simulink model "DC_Double_Closed_Loop_Speed_Regulation1"  (R2016a)
settings: Solver=VariableStepAuto  SolverMode=SingleTasking  StartTime=0  StopTime=2.5  MaxStep=1e-5  RelTol=1e-3
InitFcn:
  | run('DC_Double_Closed_Loop_Speed_Regulation.m')
values from neighbouring files (symbols this model uses):
  alpha = Un/nN    (= 0.00666666666667)    [DC_Double_Closed_Loop_Speed_Regulation.m]
  beta = Uonl/(lambda*IdN)    [DC_Double_Closed_Loop_Speed_Regulation.m]
  Ce = 0.1459    [DC_Double_Closed_Loop_Speed_Regulation.m]
  Ki = KI*taui*R/(Ks*beta)    [DC_Double_Closed_Loop_Speed_Regulation.m]    (also in motor.m = 0.5)
  Kn = (h+1)*beta*Ce*Tm/(2*h*alpha*R*Tsigman)    [DC_Double_Closed_Loop_Speed_Regulation.m]
  R = 3.68    [DC_Double_Closed_Loop_Speed_Regulation.m]    (also in motor.m = 1)
  taui = Tl    (= 0.0144)    [DC_Double_Closed_Loop_Speed_Regulation.m]
  taun = h*Tsigman    (= 0.05625)    [DC_Double_Closed_Loop_Speed_Regulation.m]
  Tl = 0.0144    [DC_Double_Closed_Loop_Speed_Regulation.m]
  Tm = 0.18    [DC_Double_Closed_Loop_Speed_Regulation.m]
  Toi = 0.0005    [DC_Double_Closed_Loop_Speed_Regulation.m]
  Ton = 0.01    [DC_Double_Closed_Loop_Speed_Regulation.m]
  Ts = 1/f    (= 0.000125)    [DC_Double_Closed_Loop_Speed_Regulation.m]
  Ucm = 5    [DC_Double_Closed_Loop_Speed_Regulation.m]
  Un = 10    [DC_Double_Closed_Loop_Speed_Regulation.m]
  Uoil = 5    [DC_Double_Closed_Loop_Speed_Regulation.m]
  Uonl = 10    [DC_Double_Closed_Loop_Speed_Regulation.m]
undefined symbols (not defined in the file or in its folder): powergui
libraries: powerlib x7, powerlib_meascontrol x1, simulink x1
settings Model: Creator=ywtyfp  LastModifiedBy=Administrator
settings DataIOCC: ReturnWorkspaceOutputs=on
settings DebuggingCC: SFUnexpectedBacktrackingDiag=error  SFNoUnconditionalDefaultTransitionDiag=error
settings SFSimCC: SimUseLocalCustomCode=on
settings RTWCC: RTWUseLocalCustomCode=on
settings GRTTargetCC: TargetLangStandard=C99 (ISO)
settings ConfigComp: CovMetricSettings=dwe  CovHtmlReporting=off  CovSaveCumulativeToWorkspaceVar=off  CovSaveSingleToWorkspaceVar=off  CovExternalEMLEnable=on

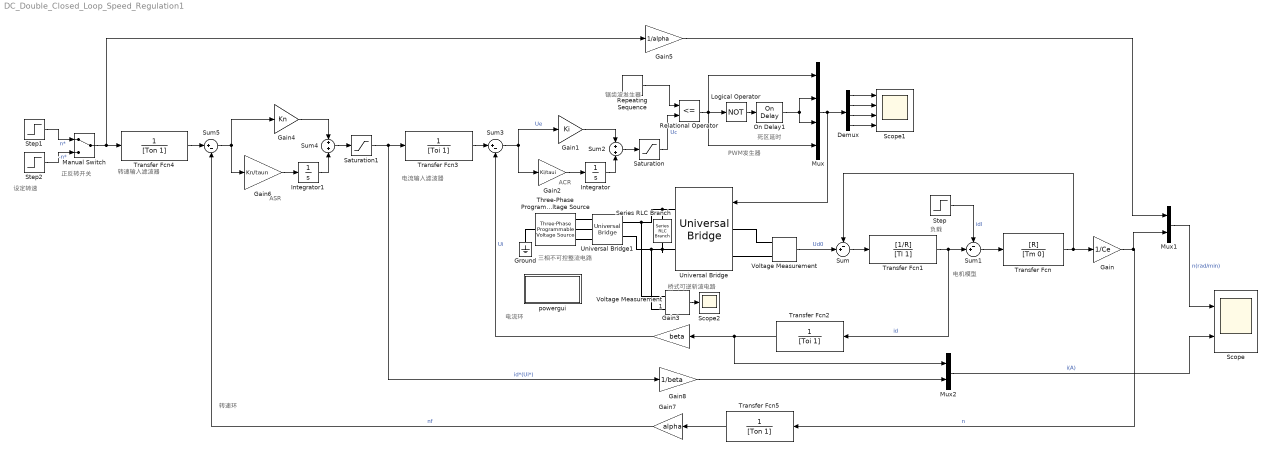
== system DC_Double_Closed_Loop_Speed_Regulation1 ==
  note: 设定转速
  note: 电流环
  note: 转速环
  note: 转速输入滤波器
  note: ASR
  note: ACR
  note: 电流输入滤波器
  note: 负载
  note: 电机模型
  note: PWM发生器
  note: 桥式可逆斩波电路
  note: 锯齿波发生器
  note: 死区延时
  note: 正反转开关
  note: 三相不可控整流电路
  Demux : Demux
  Gain : Gain  Gain=1/Ce
  Gain1 : Gain  Gain=Ki
  Gain2 : Gain  Gain=Ki/taui
  Gain3 : Gain  Gain=beta
  Gain4 : Gain  Gain=Kn
  Gain5 : Gain  Gain=1/alpha
  Gain6 : Gain  Gain=Kn/taun
  Gain7 : Gain  Gain=alpha
  Gain8 : Gain  Gain=1/beta
  Ground : powerlib/Elements/Ground  LConnTagsString=a
  Integrator : Integrator  LimitOutput=on  UpperSaturationLimit=Uoil  LowerSaturationLimit=-Uoil
  Integrator1 : Integrator  LimitOutput=on  UpperSaturationLimit=Uonl  LowerSaturationLimit=-Uonl
  Logical Operator : Logic  Operator=NOT  AllPortsSameDT=off  OutDataTypeStr=boolean
  Manual Switch : ManualSwitch
  Mux : Mux
  Mux1 : Mux  Inputs=2
  Mux2 : Mux  Inputs=2
  On Delay1 : powerlib_meascontrol/Logic/On Delay  DelayType=On delay  delay=3e-6  ic=0  Ts=0
  Relational Operator : RelationalOperator  Operator=<=  OutDataTypeStr=boolean
  Repeating Sequence : simulink/Sources/Repeating Sequence  rep_seq_t=[0 Ts]  rep_seq_y=[-Ucm Ucm]
  Saturation : Saturate  UpperLimit=Uoil  LowerLimit=-Uoil
  Saturation1 : Saturate  UpperLimit=Uonl  LowerLimit=-Uonl
  Scope : Scope  NumInputPorts=2
  Scope1 : Scope  NumInputPorts=4
  Scope2 : Scope
  Series RLC Branch : powerlib/Elements/Series RLC Branch  LConnTagsString=__new0  RConnTagsString=__new0  BranchType=C  Resistance=1  Inductance=1e-3  SetiL0=off  InitialCurrent=0  Capacitance=1e-4  Setx0=off  InitialVoltage=0  Measurements=None
  Step : Step  Time=0  After=0  SampleTime=0
  Step1 : Step  Time=0.1  After=Un  SampleTime=0
  Step2 : Step  Time=0.1  After=-Un  SampleTime=0
  Sum : Sum  Inputs=-+|
  Sum1 : Sum  Inputs=-+|
  Sum2 : Sum  Inputs=+|+
  Sum3 : Sum  Inputs=|+-
  Sum4 : Sum  Inputs=+|+
  Sum5 : Sum  Inputs=|+-
  Three-Phase Programmable Voltage Source : powerlib/Electrical Sources/Three-Phase Programmable Voltage Source  PositiveSequence="[380  0 50]"  VariationEntity=None  VariationType=Table of time-amplitude pairs  VariationTypeAlt=Step  VariationStep=0.5  VariationRate=10  VariationMagnitude=0.3  VariationFrequency=2  VariationTiming=[1 2]  VariationPhaseA=off  Amplitudes=[1 0.8 1.2 1.0]  TimeValues=[0 0.1 0.15 0.2]  HarmonicGeneration=off  HarmonicA=[3 0.2 -25 0]  HarmonicB=[2 0.15 35 2]  Timing="[0.05  3]"  BusType=swing  Pref=0  Qref=0  Qmin=-inf  Qmax=inf
  Transfer Fcn : TransferFcn  Numerator=[R]  Denominator=[Tm 0]
  Transfer Fcn1 : TransferFcn  Numerator=[1/R]  Denominator=[Tl 1]
  Transfer Fcn2 : TransferFcn  Denominator=[Toi 1]
  Transfer Fcn3 : TransferFcn  Denominator=[Toi 1]
  Transfer Fcn4 : TransferFcn  Denominator=[Ton 1]
  Transfer Fcn5 : TransferFcn  Denominator=[Ton 1]
  Universal Bridge : powerlib/Power Electronics/Universal Bridge  Arms=2  SnubberResistance=1e5  SnubberCapacitance=inf  Device=IGBT / Diodes  Ron=1e-3  Lon=0  ForwardVoltages="[  0  0  ]"  ForwardVoltage=0  GTOparameters=[ 10e-6 , 20e-6 ]  IGBTparameters=[ 1e-6 , 2e-6 ]  Measurements=None  Measurements_2=None  converterType=Rectifier
  Universal Bridge1 : powerlib/Power Electronics/Universal Bridge  Arms=3  SnubberResistance=1e5  SnubberCapacitance=inf  Device=Diodes  Ron=1e-3  Lon=0  ForwardVoltages="[  0  0  ]"  ForwardVoltage=0  GTOparameters=[ 10e-6 , 20e-6 ]  IGBTparameters=[ 1e-6 , 2e-6 ]  Measurements=None  Measurements_2=None  converterType=Rectifier
  Voltage Measurement : powerlib/Measurements/Voltage Measurement  PhasorSimulation=off  OutputType=Complex  PSBequivalent=0
  Voltage Measurement1 : powerlib/Measurements/Voltage Measurement  PhasorSimulation=off  OutputType=Complex  PSBequivalent=0
  powergui : Subsystem  Priority=1  AncestorBlock=powerlib/powergui  DialogController=POWERSYS.PowerSysDialog  InitFcn=powergui( 'InitFcn_Callback' , gcb , 0 , [ ] );  mask(PSB option menu block){SimulationMode=Continuous, SampleTime=50e-6, frequency=60, Iterations=50, frequencyindice=50, Pbase=100e6, ErrMax=1e-4, UnitsV=kV, UnitsW=MW, buscounter=0, FunctionMessages=off, echomessages=off, EnableUseOfTLC=off, CurrentSourceSwitches=off, DisableSnubberDevices=off, DisableRonSwitches=off, DisableVfSwitches=off, DisplayEquations=off, AutomaticDiscreteSolvers=off, SolverType=Tustin/Backward Euler (TBE), Interpol=off, ExternalGateDelay=off, methode=off, Ts=100, x0status=blocks, SPID=on, SwTol=0, HookPort=off, NonlinearTolerance=1e-4, nMaxIteration=100, ContinueOnMaxIteration=off, RestoreLinks=warning, ResistiveCurrentMeasurement=off, Frange=[0:2:500], Ylog=off, Xlog=on, ShowGrid=off, save=off, variable=ZData, structure=0, ZoomFFT=off, StartTime=0.0, cycles=1, DisplayStyle=1, fundamental=60, FreqAxis=off, MaxFrequency=1000, frequencyindicesteady=1, RmsSteady=1, display=off}
      mask prompts: SimulationMode "Simulation type:"; SampleTime "Sample time (s):"; frequency "Frequency (Hz):"; Iterations "Max iterations"; frequencyindice "Frequency (Hz)"; Pbase "Base power (VA)"; ErrMax "PQ tolerance (pu)"; UnitsV "Voltage units"; UnitsW "Power units"; buscounter "Load flow bus counter"; FunctionMessages "Disable Specialized Power Systems warnings"; echomessages "Display Specialized Power Systems compilation messages"; EnableUseOfTLC "Use TLC file when in Accelerator Simulation Mode and for code generation"; CurrentSourceSwitches "Disable ideal switching"; DisableSnubberDevices "Disable snubbers in switching devices"; DisableRonSwitches "Disable Ron resistances in switching devices"; DisableVfSwitches "Disable forward voltages in switching devices"; DisplayEquations "Display circuit differential equations"; AutomaticDiscreteSolvers "Automatically handle Discrete solver and Advanced tab solver settings of blocks"; SolverType "Discrete solver"; Interpol "Interpolate switching events"; ExternalGateDelay "Use time-stamped gate signals"; methode "Store switching topologies"; Ts "Buffer size (MBytes):"; x0status "Start simulation with initial electrical states from:"; SPID "Use ideal switching devices"; SwTol "Switch tolerance"; HookPort "Allow multiple powergui blocks"; NonlinearTolerance "Solver tolerance"; nMaxIteration "Maximum number of iterations"; ContinueOnMaxIteration "Continue Simulation if maximum number of iterations is reached"; RestoreLinks "Restore disabled links of Simscape Power Systems ST blocks:"; ResistiveCurrentMeasurement "Use non ideal current measurement blocks (1e-4Ohm internal resistance)"; Frange "Frequency Range"; Ylog "Log impedance"; Xlog "log Frequency"; ShowGrid "grid"; save "Save Data To Workspace"; variable "Variable Name"; structure "Structure Name (PSBFFTSCOPE)"; ZoomFFT "ZoomFFT (PSBFFTSCOPE)"; StartTime "Start Time (PSBFFTSCOPE)"; cycles "Cycles (PSBFFTSCOPE)"; DisplayStyle "Display style (PSBFFTSCOPE)"; fundamental "Fundamental (PSBFFTSCOPE)"; FreqAxis "Frequency Axis (PSBFFTSCOPE)"; MaxFrequency "Max Frequency (PSBFFTSCOPE)"; frequencyindicesteady "Frequency indice (STEADYSTATE)"; RmsSteady "RMS display (STEADYSTATE)"; display "Display Results"
      mask help: Set simulation type, simulation parameters, and preferences.
      mask init:
      | dispMessage = powergui('MaskInitialization',gcb,SimulationMode,SampleTime);
      settings: PreSaveFcn=powergui( 'PreSaveFcn_Callback' , gcb , [ ] , [ ] );  OpenFcn=sps_rtmsupport('OpenFcn',gcbh)
      mask Help: helpview(psbhelp)
      mask TypeOptions SimulationMode: Continuous | Discrete | Phasor | Discrete phasor
      mask Callback SimulationMode: powergui('SimulationType',[],[],gcb);
      mask TypeOptions UnitsV: V | kV
      mask TypeOptions UnitsW: W | kW | MW
      mask Callback CurrentSourceSwitches: powergui('SimulationType',[],[],gcb);
      mask Callback AutomaticDiscreteSolvers: powergui('SimulationType',[],[],gcb);
      mask TypeOptions SolverType: Tustin/Backward Euler (TBE) | Tustin | Backward Euler
      mask Callback SolverType: powergui('SimulationType',[],[],gcb);
      mask Callback Interpol: powergui('SimulationType',[],[],gcb);
      mask Callback ExternalGateDelay: powergui('SimulationType',[],[],gcb);
      mask Callback methode: powergui('SimulationType',[],[],gcb);
      mask TypeOptions x0status: blocks | steady | zero
      mask TypeOptions RestoreLinks: yes | warning | no
      mask Callback display: sps_rtmsupport('parametereditingmodes',gcbh) % Will be executed last in parameter callbacks to ensure mask enable consistency
      mask DialogControl AutoSolverNote Prompt: The Simulation type parameter is governed by Simulink. To access the Powergui solver settings, unselect auto (Automatic solver selection) solver in the Simulink solver options.
      mask DialogControl SteadyState Prompt: Steady-State
      mask DialogControl SteadyState Callback:
      | close_system(gcb)
      | power_steadystate(bdroot(gcb),gcb);
      mask DialogControl InitialState Prompt: Initial State
      mask DialogControl InitialState Callback:
      | close_system(gcb)
      | power_initstates(bdroot(gcb),gcb)
      mask DialogControl MachineInitialization Prompt: Machine Initialization
      mask DialogControl MachineInitialization Callback:
      | close_system(gcb)
      | power_loadflow(bdroot(gcb),gcb)
      mask DialogControl ImpedanceMeasurement Prompt: Impedance Measurement
      mask DialogControl ImpedanceMeasurement Callback:
      | close_system(gcb)
      | power_zmeter(bdroot(gcb),gcb)
      mask DialogControl FFTAnalysis Prompt: FFT Analysis
      mask DialogControl FFTAnalysis Callback:
      | close_system(gcb)
      | power_fftscope(bdroot(gcb),gcb)
      mask DialogControl LinearSystemAnalyzer Prompt: Use Linear System Analyzer
      mask DialogControl LinearSystemAnalyzer Callback:
      | close_system(gcb)
      | power_ltiview(bdroot(gcb),gcb)
      mask DialogControl HysteresisDesign Prompt: Hysteresis Design
      mask DialogControl HysteresisDesign Callback:
      | close_system(gcb)
      | power_hysteresis(bdroot(gcb),gcb)
      mask DialogControl RLCLineParameters Prompt: RLC Line Parameters
      mask DialogControl RLCLineParameters Callback:
      | close_system(gcb)
      | power_lineparam(bdroot(gcb),gcb)
      mask DialogControl GenerateReprot Prompt: Generate Report
      mask DialogControl GenerateReprot Callback:
      | close_system(gcb)
      | power_report(bdroot(gcb),gcb)
      mask DialogControl Control14 Prompt: Customize SPS blocks
      mask DialogControl Control14 Callback:
      | close_system(gcb);
      | power_customize;
      mask DialogControl LoadFlow Prompt: Load Flow
      mask DialogControl LoadFlow Callback:
      | close_system(gcb)
      | power_loadflow('-v2',bdroot(gcb))
      mask DialogControl Container14 Prompt: Load flow settings
      mask DialogControl Solver Prompt: Solver
      mask DialogControl SolverDetails Prompt: Solver details for nonlinear elements
      mask Display: color('blue'),disp(dispMessage)
  wires:
  Sum/1 -> Transfer Fcn1/1
  Sum1/1 -> Transfer Fcn/1
  Transfer Fcn/1 -> Sum/1, Gain/1
  Gain/1 -> Mux1/2, Transfer Fcn5/1  "n"
  Step/1 -> Sum1/1  "idl"
  Voltage Measurement/1 -> Sum/2  "Ud0"
  Repeating Sequence/1 -> Relational Operator/1
  Mux/1 -> Demux/1, Universal Bridge/1
  Gain2/1 -> Integrator/1
  Saturation/1 -> Relational Operator/2  "Uc"
  Integrator/1 -> Sum2/2
  Sum2/1 -> Saturation/1
  Gain1/1 -> Sum2/1
  Transfer Fcn2/1 -> Mux2/1, Gain3/1
  Transfer Fcn1/1 -> Transfer Fcn2/1, Sum1/2  "id"
  Gain3/1 -> Sum3/2  "Ui"
  Sum3/1 -> Gain2/1, Gain1/1  "Ue"
  Transfer Fcn3/1 -> Sum3/1
  Gain4/1 -> Sum4/1
  Sum4/1 -> Saturation1/1
  Integrator1/1 -> Sum4/2
  Gain6/1 -> Integrator1/1
  Saturation1/1 -> Transfer Fcn3/1, Gain8/1  "id*(Ui*)"
  Transfer Fcn5/1 -> Gain7/1
  Gain7/1 -> Sum5/2  "nf"
  Sum5/1 -> Gain6/1, Gain4/1
  Transfer Fcn4/1 -> Sum5/1
  Mux1/1 -> Scope/1  "n(rad/min)"
  Gain5/1 -> Mux1/1
  Mux2/1 -> Scope/2  "i(A)"
  Relational Operator/1 -> Mux/4, Mux/1, Logical Operator/1
  Demux/3 -> Scope1/3
  Demux/4 -> Scope1/4
  Demux/2 -> Scope1/2
  Demux/1 -> Scope1/1
  Logical Operator/1 -> On Delay1/1
  Gain8/1 -> Mux2/2
  Voltage Measurement1/1 -> Scope2/1
  On Delay1/1 -> Mux/2, Mux/3
  Manual Switch/1 -> Gain5/1, Transfer Fcn4/1
  Step1/1 -> Manual Switch/1  "n*"
  Step2/1 -> Manual Switch/2  "-n*"
  connections:
  Universal Bridge1/RConn1 -- Series RLC Branch/LConn1 -- Universal Bridge/RConn1 -- Voltage Measurement1/LConn1
  Universal Bridge1/RConn2 -- Voltage Measurement1/LConn2 -- Series RLC Branch/RConn1 -- Universal Bridge/RConn2
  Universal Bridge/LConn1 -- Voltage Measurement/LConn1
  Universal Bridge/LConn2 -- Voltage Measurement/LConn2
  Three-Phase Programmable Voltage Source/LConn1 -- Ground/LConn1
  Three-Phase Programmable Voltage Source/RConn3 -- Universal Bridge1/LConn3
  Three-Phase Programmable Voltage Source/RConn2 -- Universal Bridge1/LConn2
  Three-Phase Programmable Voltage Source/RConn1 -- Universal Bridge1/LConn1

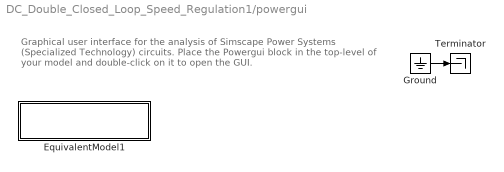
== system DC_Double_Closed_Loop_Speed_Regulation1/powergui ==
  note: Graphical user interface for the analysis of
      | Simscape Power Systems (Specialized Technology) circuits.
      | Place the Powergui block in the top-level of your model and double-click
      | on it to open the GUI.
  EquivalentModel1 : Subsystem  mask{SwTol=SwTol}
      mask prompts: SwTol "SwitchTolerance"
      mask init:
      | S  = GetDataForEquivalentModel('SPID',gcbh,SwTol);
      mask Display:
      | color('blue')
      | disp('EQUIVALENT CIRCUIT\nSPID')
  Ground : Ground
  Terminator : Terminator
  wires:
  Ground/1 -> Terminator/1

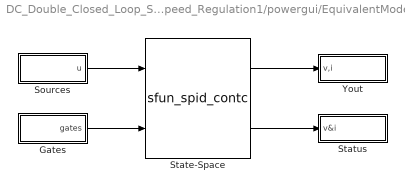
== system DC_Double_Closed_Loop_Speed_Regulation1/powergui/EquivalentModel1 ==
  Gates : Subsystem
  Sources : Subsystem
  State-Space : S-Function  FunctionName=sfun_spid_contc  Parameters=S.Mg, [S.nb.x S.nb.u S.nb.y S.nb.s], S.x0, S.MgColNames, S.SwitchVf, S.SwitchType, S.SwitchGateInitialValue, S.SwitchTolerance,S.SaveMatrices,S.BufferSize  SFunctionDeploymentMode=off  EnableBusSupport=off
  Status : Subsystem
  Yout : Subsystem
  wires:
  State-Space/1 -> Yout/1(v,i)
  State-Space/2 -> Status/1(v&i)
  Gates/1(gates) -> State-Space/2
  Sources/1(u) -> State-Space/1

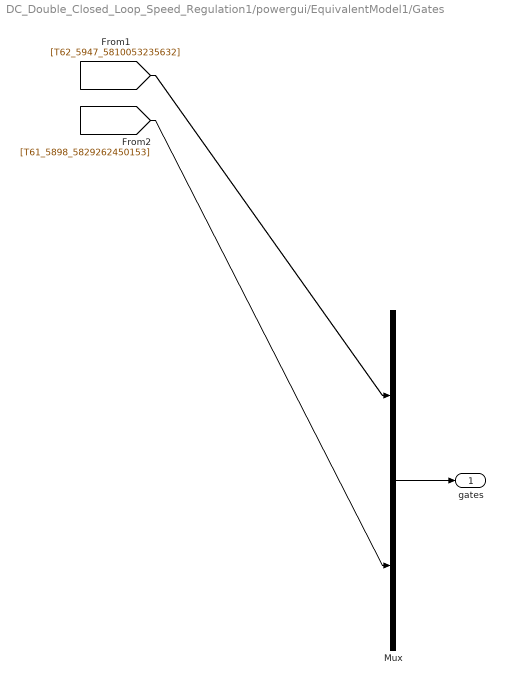
== system DC_Double_Closed_Loop_Speed_Regulation1/powergui/EquivalentModel1/Gates ==
  Mux : Mux  Inputs=[6 4]
  gates : Outport
  wires:
  Mux/1 -> gates/1
  [T62_5947_5810053235632] -> Mux/1
  [T61_5898_5829262450153] -> Mux/2

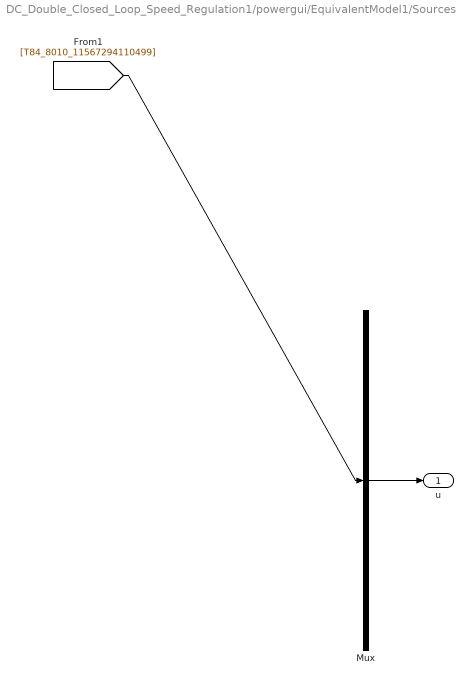
== system DC_Double_Closed_Loop_Speed_Regulation1/powergui/EquivalentModel1/Sources ==
  Mux : Mux  Inputs=1
  u : Outport
  wires:
  Mux/1 -> u/1
  [T84_8010_11567294110499] -> Mux/1

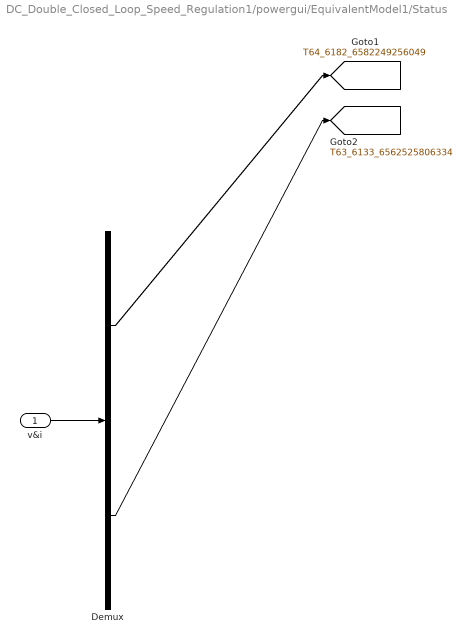
== system DC_Double_Closed_Loop_Speed_Regulation1/powergui/EquivalentModel1/Status ==
  v&i : Inport
  Demux : Demux  Outputs=[12 8]
  tag scope: T63_6133_6562525806334=global, T64_6182_6582249256049=global
  wires:
  v&i/1 -> Demux/1
  Demux/1 -> [T64_6182_6582249256049]
  Demux/2 -> [T63_6133_6562525806334]

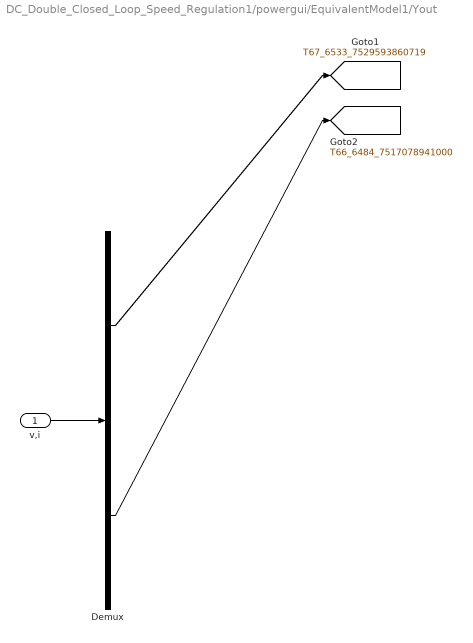
== system DC_Double_Closed_Loop_Speed_Regulation1/powergui/EquivalentModel1/Yout ==
  v,i : Inport
  Demux : Demux  Outputs=[1 1]
  tag scope: T66_6484_7517078941000=global, T67_6533_7529593860719=global
  wires:
  v,i/1 -> Demux/1
  Demux/1 -> [T67_6533_7529593860719]
  Demux/2 -> [T66_6484_7517078941000]
